simulink model "Filtro_EMA_Sensor_Laser"  (R2022b)
settings: Solver=VariableStepAuto  StartTime=0.0  StopTime=0.2  RelTol=1e-3
undefined symbols (not defined in the file): x
settings Model: Creator=rafa-  LastModifiedBy=rafa-

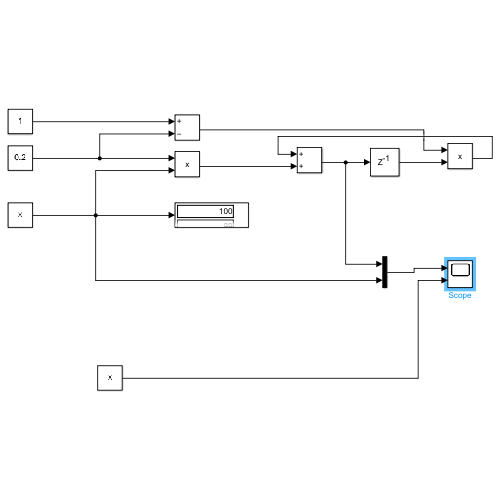
[thumbnail: Simulink's stored preview of the top-level diagram]
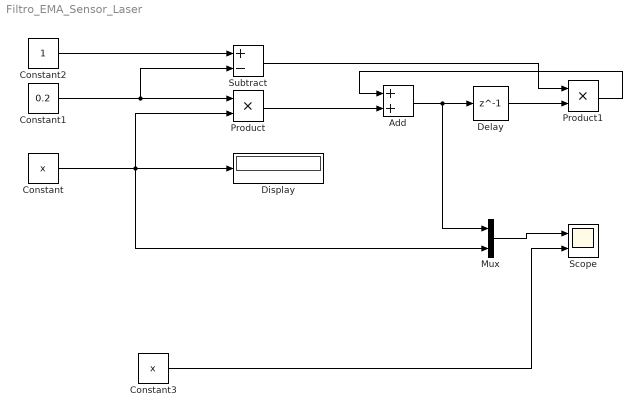
== system Filtro_EMA_Sensor_Laser ==
  Add : Sum
  Constant : Constant  Value=x
  Constant1 : Constant  Value=0.2
  Constant2 : Constant
  Constant3 : Constant  Value=x
  Delay : Delay  DelayLength=1  InitialCondition=0
  Display : Display
  Mux : Mux  Inputs=2
  Product : Product
  Product1 : Product
  Scope : Scope  NumInputPorts=2
  Subtract : Sum  Inputs=+-
  wires:
  Constant2/1 -> Subtract/1
  Constant1/1 -> Subtract/2, Product/1
  Constant/1 -> Mux/2, Product/2, Display/1
  Product/1 -> Add/2
  Add/1 -> Mux/1, Delay/1
  Delay/1 -> Product1/2
  Subtract/1 -> Product1/1
  Product1/1 -> Add/1
  Mux/1 -> Scope/1
  Constant3/1 -> Scope/2
